simulink model "MoPhong"  (R2023a)
settings: Solver=VariableStepAuto  StartTime=0.0  StopTime=10.0  RelTol=1e-3
values from neighbouring files (symbols this model uses):
  DL = 2*psi*sqrt(JL*KL)    [Code.m]
  JL = NL*Jm    (= 0.112)    [Code.m]
  Jm = 0.014    [Code.m]
  KL = 225    [Code.m]
  Kp = cp*wL    [Code.m]
  Kvg = Kv*(Jm+JL/Ng^2)    [Code.m]
  Ng = 1    [Code.m]
  position = 7    [Code.m]
  velocity = 7    [Code.m]
libraries: simulink x1
settings Model: Creator=admin  LastModifiedBy=admin

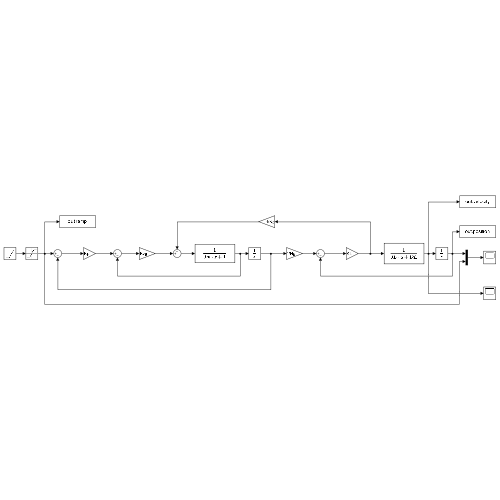
[thumbnail: Simulink's stored preview of the top-level diagram]
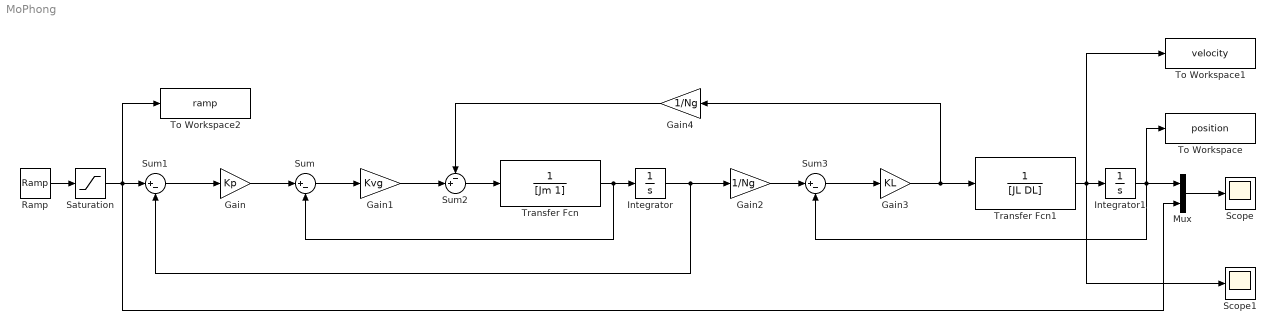
== system MoPhong ==
  Gain : Gain  Gain=Kp
  Gain1 : Gain  Gain=Kvg
  Gain2 : Gain  Gain=1/Ng
  Gain3 : Gain  Gain=KL
  Gain4 : Gain  Gain=1/Ng
  Integrator : Integrator
  Integrator1 : Integrator
  Mux : Mux  Inputs=2
  Ramp : simulink/Sources/Ramp  slope=velocity  start=0  InitialOutput=0
  Saturation : Saturate  UpperLimit=position  LowerLimit=0
  Scope : Scope
  Scope1 : Scope
  Sum : Sum  Inputs=|+-
  Sum1 : Sum  Inputs=|+-
  Sum2 : Sum  Inputs=-+|
  Sum3 : Sum  Inputs=|+-
  To Workspace : ToWorkspace  VariableName=position  SaveFormat=Timeseries  SampleTime=-1
  To Workspace1 : ToWorkspace  VariableName=velocity  SaveFormat=Timeseries  SampleTime=-1
  To Workspace2 : ToWorkspace  VariableName=ramp  SaveFormat=Timeseries  SampleTime=-1
  Transfer Fcn : TransferFcn  Denominator=[Jm 1]
  Transfer Fcn1 : TransferFcn  Denominator=[JL DL]
  wires:
  Sum2/1 -> Transfer Fcn/1
  Gain2/1 -> Sum3/1
  Sum3/1 -> Gain3/1
  Gain3/1 -> Gain4/1, Transfer Fcn1/1
  Transfer Fcn1/1 -> To Workspace1/1, Scope1/1, Integrator1/1
  Sum1/1 -> Gain/1
  Gain/1 -> Sum/1
  Sum/1 -> Gain1/1
  Gain1/1 -> Sum2/2
  Transfer Fcn/1 -> Integrator/1, Sum/2
  Integrator/1 -> Sum1/2, Gain2/1
  Gain4/1 -> Sum2/1
  Integrator1/1 -> Mux/1, Sum3/2, To Workspace/1
  Saturation/1 -> To Workspace2/1, Sum1/1, Mux/2
  Mux/1 -> Scope/1
  Ramp/1 -> Saturation/1
